simulink model "PI_Laengsregler_2"  (R2019b)
settings: Solver=VariableStepAuto  StartTime=0.0  StopTime=20  FixedStep=1e-6  MaxStep=1e-4  RelTol=1e-3
values from neighbouring files (symbols this model uses):
  A = [a11, a12, a13, a14, a15; a21, a22, a23, a24, a25; a31, a32, a33, a34,     a35; a41, a42, a43, a44, a45; a51, a52, a53, a54, a55]    [initial_data.m]
undefined symbols (not defined in the file or in its folder): b, cT, tau
libraries: simulink x2, cstblocks x1

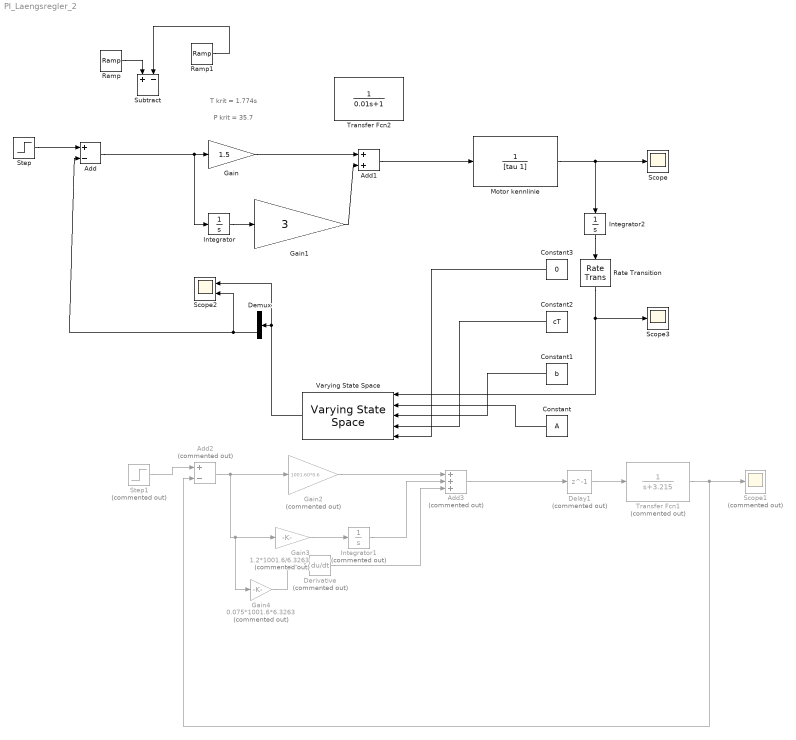
== system PI_Laengsregler_2 ==
  note: T krit = 1.774s
  note: P krit = 35.7
  Add : Sum  Inputs=+-
  Add1 : Sum
  Add2 : Sum  Commented=on  Inputs=+-
  Add3 : Sum  Commented=on  Inputs=+++
  Constant : Constant  Value=A  VectorParams1D=off
  Constant1 : Constant  Value=b  VectorParams1D=off
  Constant2 : Constant  Value=cT  VectorParams1D=off
  Constant3 : Constant  Value=0
  Delay1 : Delay  Commented=on  DelayLength=1
  Demux : Demux  Outputs=2
  Derivative : Derivative  Commented=on
  Gain : Gain  Gain=1.5
  Gain1 : Gain  Gain=3
  Gain2 : Gain  Commented=on  Gain=1001.60*0.6
  Gain3 : Gain  Commented=on  Gain=1.2*1001.6/6.3263
  Gain4 : Gain  Commented=on  Gain=0.075*1001.6*6.3263
  Integrator : Integrator
  Integrator1 : Integrator  Commented=on
  Integrator2 : Integrator
  Motor kennlinie : TransferFcn  Denominator=[tau 1]
  Ramp : simulink/Sources/Ramp  slope=1  start=0  InitialOutput=0
  Ramp1 : simulink/Sources/Ramp  slope=1  start=1  InitialOutput=0
  Rate Transition : RateTransition  OutPortSampleTime=tasten
  Scope : Scope
  Scope1 : Scope  Commented=on
  Scope2 : Scope  NumInputPorts=2
  Scope3 : Scope
  Step : Step  SampleTime=0
  Step1 : Step  Commented=on  SampleTime=0
  Subtract : Sum  Inputs=+-
  Transfer Fcn1 : TransferFcn  Commented=on  Denominator=[1 3.215]
  Transfer Fcn2 : TransferFcn  Denominator=[0.01 1]
  Varying State Space : cstblocks/Linear Parameter Varying/Varying State Space  x0=0  xNames=''  OutputX=on  OutputDX=on
  wires:
  Transfer Fcn1/1 -> Add2/2, Scope1/1
  Add3/1 -> Delay1/1
  Gain3/1 -> Integrator1/1
  Step1/1 -> Add2/1
  Gain2/1 -> Add3/1
  Add2/1 -> Gain4/1, Gain3/1, Gain2/1
  Delay1/1 -> Transfer Fcn1/1
  Gain4/1 -> Derivative/1
  Integrator1/1 -> Add3/2
  Derivative/1 -> Add3/3
  Add/1 -> Integrator/1, Gain/1
  Gain/1 -> Add1/1
  Integrator/1 -> Gain1/1
  Ramp/1 -> Subtract/1
  Ramp1/1 -> Subtract/2
  Demux/2 -> Scope2/2, Add/2
  Constant2/1 -> Varying State Space/4
  Constant/1 -> Varying State Space/2
  Constant3/1 -> Varying State Space/5
  Constant1/1 -> Varying State Space/3
  Integrator2/1 -> Rate Transition/1
  Varying State Space/2 -> Scope2/1, Demux/1
  Step/1 -> Add/1
  Rate Transition/1 -> Varying State Space/1, Scope3/1
  Gain1/1 -> Add1/2
  Add1/1 -> Motor kennlinie/1
  Motor kennlinie/1 -> Scope/1, Integrator2/1
